simulink model "io301"  (Simulink 6.0)
settings: Solver=ode5  StartTime=0.0  StopTime=0.2  FixedStep=0.001  RelTol=1e-3
libraries: xpcdiamondlib x4
settings Model: Creator=ekbas  LastModifiedBy=ekbas  ExtModeArmWhenConnect=off  BufferReuse=off
settings DataIOCC: SaveFormat=Structure  SignalLoggingName=sigsOut
settings OptimizationCC: InlineInvariantSignals=off  OptimizeBlockIOStorage=off  BufferReuse=off  EnforceIntegerDowncast=off  FoldNonRolledExpr=off  LocalBlockOutputs=off
settings DebuggingCC: CheckExecutionContextPreStartOutputMsg=on  CheckExecutionContextRuntimeOutputMsg=on  SolverPrmCheckMsg=none
settings RTWCC: SystemTargetFile=xpctarget.tlc  TemplateMakefile=xpc_default_tmf  ProcessScript=xpctarget_make_rtw_hook
settings xpcTargetCC: TargetFcnLib=ansi_tfl_tmw.mat  GenFloatMathFcnCalls=ANSI_C  ModelReferenceCompliant=off  LifeSpan=inf
settings SFSimCC: SFSimApplyToAllLibs=on  SFSimBuildMode=Incremental

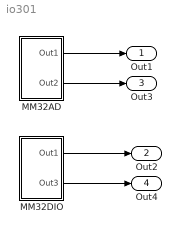
== system io301 ==
  MM32AD : Subsystem  PropExecContextAcrossSSBoundary=on
  MM32DIO : Subsystem  PropExecContextAcrossSSBoundary=on
  Out1 : Outport
  Out2 : Outport  Port=2
  Out3 : Outport  Port=3
  Out4 : Outport  Port=4
  wires:
  MM32AD/1(Out1) -> Out1/1
  MM32DIO/1(Out1) -> Out2/1
  MM32AD/2(Out2) -> Out3/1
  MM32DIO/2(Out3) -> Out4/1

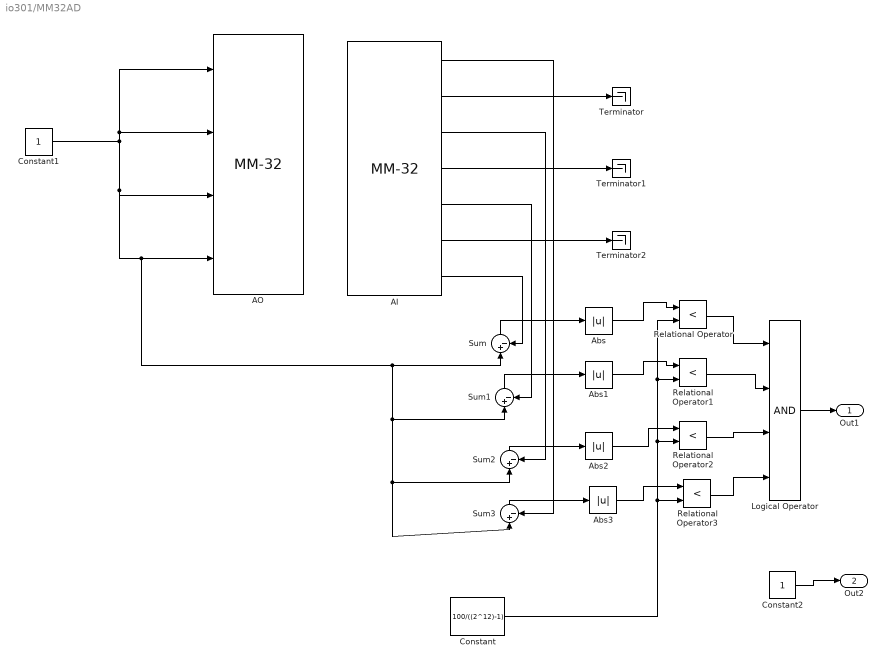
== system io301/MM32AD ==
  AI : xpcdiamondlib/A//D/MM-32   configuration=1-16 DI  firstChan=1  numChans=7  range=-10V to +10V  sampleTime=0.001  base=0x280
  AO : xpcdiamondlib/D//A/MM-32   channel=[1 2 3 4]  range=+-10V  reset=[1]  initValue=[0]  sampletime=0.001  baseaddress=0x280
  Abs{,1..3} (4 alike) : Abs  SaturateOnIntegerOverflow=on
  Constant : Constant  Value=100/((2^12)-1)
  Constant1 : Constant
  Constant2 : Constant
  Logical Operator : Logic  Inputs=4  AllPortsSameDT=off
  Relational Operator{,1..3} (4 alike) : RelationalOperator  Operator=<
  Sum{,1..3} (4 alike) : Sum  Orientation=up  Inputs=|+-  SaturateOnIntegerOverflow=on
  Terminator : Terminator
  Terminator1 : Terminator
  Terminator2 : Terminator
  Out1 : Outport
  Out2 : Outport  Port=2
  wires:
  Constant1/1 -> AO/1, AO/2, AO/3, AO/4, Sum/1, Sum1/1, Sum2/1, Sum3/1
  AI/1 -> Sum3/2
  Sum/1 -> Abs/1
  Sum1/1 -> Abs1/1
  Sum2/1 -> Abs2/1
  Sum3/1 -> Abs3/1
  Constant/1 -> Relational Operator3/2, Relational Operator2/2, Relational Operator1/2, Relational Operator/2
  Abs3/1 -> Relational Operator3/1
  Abs/1 -> Relational Operator/1
  Abs1/1 -> Relational Operator1/1
  Abs2/1 -> Relational Operator2/1
  Relational Operator/1 -> Logical Operator/1
  Relational Operator1/1 -> Logical Operator/2
  Relational Operator2/1 -> Logical Operator/3
  Relational Operator3/1 -> Logical Operator/4
  AI/7 -> Sum/2
  AI/3 -> Sum2/2
  AI/5 -> Sum1/2
  AI/2 -> Terminator/1
  AI/6 -> Terminator2/1
  AI/4 -> Terminator1/1
  Logical Operator/1 -> Out1/1
  Constant2/1 -> Out2/1

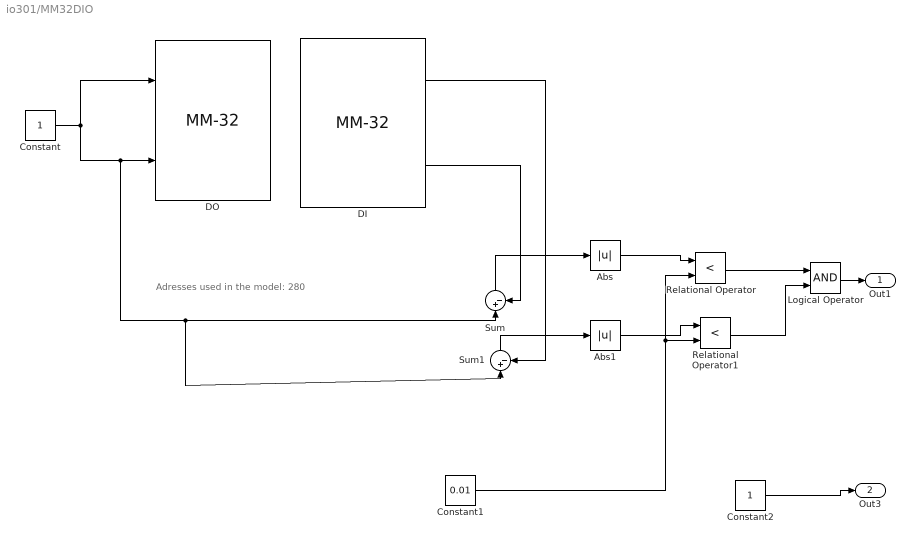
== system io301/MM32DIO ==
  note: Adresses used in the model: 280
  Abs : Abs  SaturateOnIntegerOverflow=on
  Abs1 : Abs  SaturateOnIntegerOverflow=on
  Constant : Constant
  Constant1 : Constant  Value=0.01
  Constant2 : Constant
  DI : xpcdiamondlib/Digital Input/MM-32   channel=[1,5]  port=B  chip=1  sampletime=0.001  baseaddress=0x280
  DO : xpcdiamondlib/Digital Output/MM-32   channel=[1,5]  port=C  reset=[1]  initValue=[0]  chip=1  sampletime=0.001  baseaddress=0x280
  Logical Operator : Logic  AllPortsSameDT=off
  Relational Operator : RelationalOperator  Operator=<
  Relational Operator1 : RelationalOperator  Operator=<
  Sum : Sum  Orientation=up  Inputs=|+-  SaturateOnIntegerOverflow=on
  Sum1 : Sum  Orientation=up  Inputs=|+-  SaturateOnIntegerOverflow=on
  Out1 : Outport
  Out3 : Outport  Port=2
  wires:
  Abs1/1 -> Relational Operator1/1
  Constant1/1 -> Relational Operator/2, Relational Operator1/2
  DI/2 -> Sum/2
  DI/1 -> Sum1/2
  Relational Operator/1 -> Logical Operator/1
  Abs/1 -> Relational Operator/1
  Sum1/1 -> Abs1/1
  Sum/1 -> Abs/1
  Constant/1 -> Sum1/1, Sum/1, DO/2, DO/1
  Relational Operator1/1 -> Logical Operator/2
  Logical Operator/1 -> Out1/1
  Constant2/1 -> Out3/1
